simulink model "project_2023_11_6_p48"  (R2017b)
settings: Solver=VariableStepAuto  StartTime=0.0  StopTime=0.1  RelTol=1e-3
settings Model: Creator=Administrator  LastModifiedBy=Administrator
settings SolverCC: MaxConsecutiveMinStep=0.01

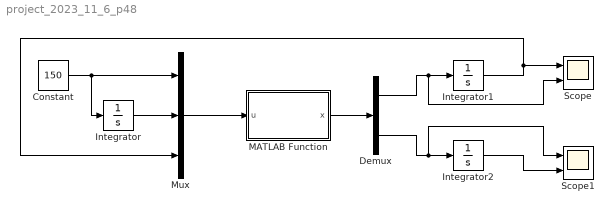
== system project_2023_11_6_p48 ==
  Constant : Constant  Value=150
  Demux : Demux  Outputs=2
  Integrator : Integrator
  Integrator1 : Integrator
  Integrator2 : Integrator
  MATLAB Function : MATLAB Function  TreatAsAtomicUnit=on
  Mux : Mux  Inputs=3
  Scope : Scope  NumInputPorts=2
  Scope1 : Scope  NumInputPorts=2
  wires:
  Constant/1 -> Integrator/1, Mux/1
  Integrator/1 -> Mux/2
  Mux/1 -> MATLAB Function/1(u)
  MATLAB Function/1(x) -> Demux/1
  Demux/1 -> Scope/2, Integrator1/1
  Demux/2 -> Scope1/1, Integrator2/1
  Integrator1/1 -> Mux/3, Scope/1
  Integrator2/1 -> Scope1/2

== matlab function project_2023_11_6_p48/MATLAB Function ==
  data: u input; x output
function x   = compv(u)
%参数说明：r1 曲柄长度，r2 连杆长度
%u(1)曲柄角速度; u(2)曲柄角度; u(3)连杆角度
r1 = 15;  r2 = 55;
a = [r2 * sin(u(3)) 1;r2 * cos(u(3)) 0];
b = -u(1) * r1 * [sin(u(2)); cos(u(2))];

x = inv(a) * b;
